simulink model "TP2Asintotico"  (R2024b)
settings: Solver=VariableStepAuto  StartTime=0.0  StopTime=10.0  FixedStep=0.  RelTol=1e-3
values from neighbouring files (symbols this model uses):
  D = 0    [DatosModelo.m]    (also in EstimadorAsintotico.m = 0.08; EstimadorExponencial.m = 0.08; EstimadorKalman.m = 0.08)
  F = zeros(length(modelParameters.K),1)    [DatosModelo.m]
  n0 = 100    [DatosModelo.m]    (also in EstimadorAsintotico.m = 0; EstimadorExponencial.m = 0; EstimadorKalman.m = 0)
  p0 = 0    [DatosModelo.m]    (also in EstimadorAsintotico.m; EstimadorExponencial.m; EstimadorKalman.m)
  Q = zeros(length(modelParameters.K),1)    [DatosModelo.m]
  s0 = 50    [DatosModelo.m]    (also in EstimadorAsintotico.m = 1; EstimadorExponencial.m = 1; EstimadorKalman.m = 1)
  v0 = 1    [DatosModelo.m]
  x0 = 1    [DatosModelo.m]    (also in EstimadorAsintotico.m = 5; EstimadorExponencial.m = 5; EstimadorKalman.m = 5)
  xi_in = [x0; s0; n0; p0]    [EstimadorAsintotico.m]    (also in EstimadorExponencial.m; EstimadorKalman.m)
  z0 = s0*1.5    (= 1.5)    [EstimadorAsintotico.m]
undefined symbols (not defined in the file or in its folder): sustratePerturbance
settings Model: Creator=tomii  LastModifiedBy=tomii

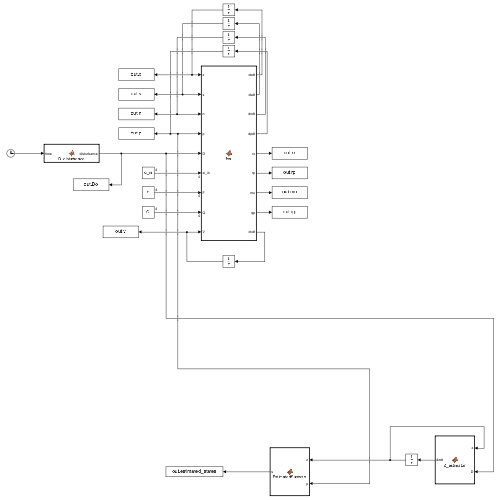
[thumbnail: Simulink's stored preview of the top-level diagram]
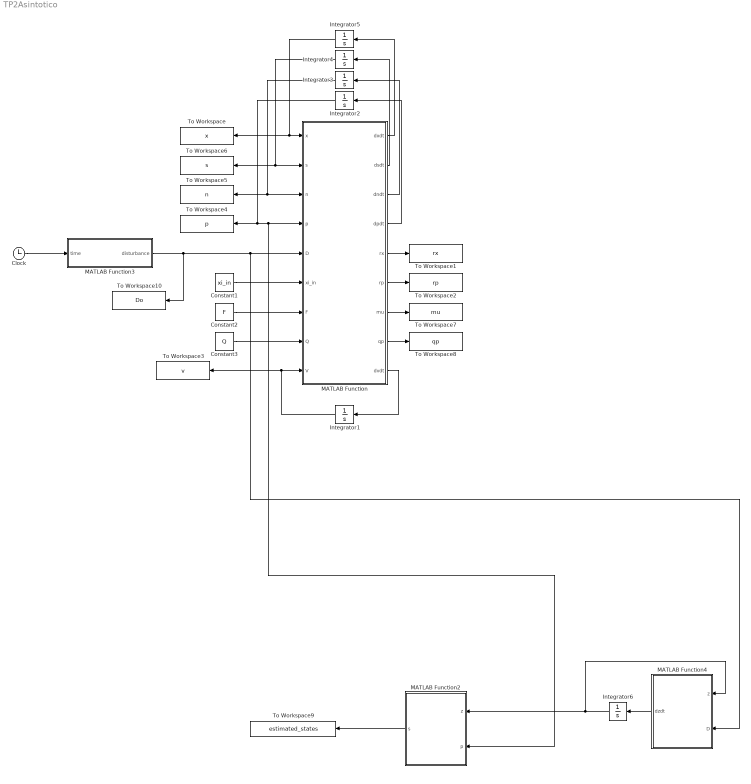
== system TP2Asintotico ==
  Clock : Clock
  Constant1 : Constant  Value=xi_in
  Constant2 : Constant  Value=F
  Constant3 : Constant  Value=Q
  Integrator1 : Integrator  InitialCondition=v0
  Integrator2 : Integrator  InitialCondition=p0
  Integrator3 : Integrator  InitialCondition=n0
  Integrator4 : Integrator  InitialCondition=s0
  Integrator5 : Integrator  InitialCondition=x0
  Integrator6 : Integrator  InitialCondition=z0
  MATLAB Function : MATLAB Function  TreatAsAtomicUnit=on
  MATLAB Function2 : MATLAB Function  TreatAsAtomicUnit=on
  MATLAB Function3 : MATLAB Function  TreatAsAtomicUnit=on
  MATLAB Function4 : MATLAB Function  TreatAsAtomicUnit=on
  To Workspace : ToWorkspace  VariableName=x  SaveFormat=Timeseries  SampleTime=-1
  To Workspace1 : ToWorkspace  VariableName=rx  SaveFormat=Timeseries  SampleTime=-1
  To Workspace10 : ToWorkspace  VariableName=Do  SaveFormat=Timeseries  SampleTime=-1
  To Workspace2 : ToWorkspace  VariableName=rp  SaveFormat=Timeseries  SampleTime=-1
  To Workspace3 : ToWorkspace  VariableName=v  SaveFormat=Timeseries  SampleTime=-1
  To Workspace4 : ToWorkspace  VariableName=p  SaveFormat=Timeseries  SampleTime=-1
  To Workspace5 : ToWorkspace  VariableName=n  SaveFormat=Timeseries  SampleTime=-1
  To Workspace6 : ToWorkspace  VariableName=s  SaveFormat=Timeseries  SampleTime=-1
  To Workspace7 : ToWorkspace  VariableName=mu  SaveFormat=Timeseries  SampleTime=-1
  To Workspace8 : ToWorkspace  VariableName=qp  SaveFormat=Timeseries  SampleTime=-1
  To Workspace9 : ToWorkspace  VariableName=estimated_states  SaveFormat=Timeseries  SampleTime=-1
  wires:
  Constant1/1 -> MATLAB Function/6(xi_in)
  Constant2/1 -> MATLAB Function/7(F)
  Constant3/1 -> MATLAB Function/8(Q)
  MATLAB Function/5(rx) -> To Workspace1/1
  MATLAB Function/6(rp) -> To Workspace2/1
  MATLAB Function/9(dvdt) -> Integrator1/1
  Integrator1/1 -> MATLAB Function/9(V), To Workspace3/1
  MATLAB Function/1(dxdt) -> Integrator5/1
  MATLAB Function/2(dsdt) -> Integrator4/1
  MATLAB Function/3(dndt) -> Integrator3/1
  MATLAB Function/4(dpdt) -> Integrator2/1
  Integrator2/1 -> To Workspace4/1, MATLAB Function2/2(p), MATLAB Function/4(p)
  Integrator3/1 -> To Workspace5/1, MATLAB Function/3(n)
  MATLAB Function/7(mu) -> To Workspace7/1
  MATLAB Function/8(qp) -> To Workspace8/1
  MATLAB Function2/1(s) -> To Workspace9/1
  Integrator5/1 -> To Workspace/1, MATLAB Function/1(x)
  Integrator4/1 -> MATLAB Function/2(s), To Workspace6/1
  MATLAB Function3/1(disturbance) -> To Workspace10/1, MATLAB Function4/2(D), MATLAB Function/5(D)
  Clock/1 -> MATLAB Function3/1(time)
  MATLAB Function4/1(dzdt) -> Integrator6/1
  Integrator6/1 -> MATLAB Function2/1(z), MATLAB Function4/1(z)

== matlab function TP2Asintotico/MATLAB Function ==
  data: dxdt output; dsdt output; dndt output; dpdt output; x input; s input; n input; p input; D input; xi_in input; F input; Q input; V input; modelParameters parameter; rx output; rp output; mu output; qp output; dvdt output
function [dxdt, dsdt, dndt, dpdt, rx, rp, mu, qp, dvdt] = fcn(x, s, n, p, D, xi_in, F, Q, V, modelParameters)   
    % Modelo de Monod
    rx_params=modelParameters.rx_params;
    rp_params=modelParameters.rp_params;
    Kipn=modelParameters.Kipn;
    K=modelParameters.K;
    
    mu=HaldaneMonodModel(s, n, rx_params);
    qp=HaldaneMonodModel(s, n, rp_params);
    rx=mu*n;
    rp=qp*Kipn;

    states = K * [rx;rp] * x + ([0;D*(xi_in(2)-s);D*(xi_in(3)-n);0]) + F - Q;
    % states = K * [rx;rp] * x + (xi_in-[x;s;n;p]*[1,1])*[1;1]*D + F - Q;
    dvdt = D*V;

    dxdt=states(1);
    dsdt=states(2);
    dndt=states(3);
    dpdt=states(4);
end

== matlab function TP2Asintotico/MATLAB Function2 ==
  data: z input; p input; s output; params parameter
function s = EstimatedSustrate(z, p, params)

    Ks2 = params.Ks2;

    s = -z+Ks2*p;

end

== matlab function TP2Asintotico/MATLAB Function3 ==
  data: time input; disturbance output; sustratePerturbance parameter; D parameter
function disturbance = D_disturbance(time, sustratePerturbance, D)

disturbancePercentage = sustratePerturbance.disturbancePercentage;
perturbanceStart = sustratePerturbance.perturbanceStart;
perturbanceStop = sustratePerturbance.perturbanceStop;

if (time > perturbanceStart) && (time < perturbanceStop)
% if (triggeredFlag == 0) && (time > perturbanceStart)
    disturbance = (disturbancePercentage/100+1)*D;
else
   disturbance = 0;
end

== matlab function TP2Asintotico/MATLAB Function4 ==
  data: z input; dzdt output; D input; params parameter
function dzdt = Z_estimator(z, D, params)
    
    s_in = params.s_in;
    Ks2 = params.Ks2;

    dzdt = -D*z+Ks2*D*s_in;
    % dzdt = D*(ks2*p+s_in-s)

end
